simulink subsystem "Map_to_queue"  (R2020a)
settings: Solver=VariableStepAuto  StartTime=0.0  StopTime=10.0  RelTol=1e-3
libraries: simulink x1
settings Model: Creator=zinoex  LastModifiedBy=zinoex

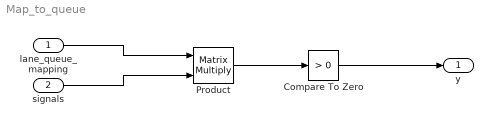
== system Map_to_queue ==
  lane_queue_mapping : Inport
  signals : Inport  Port=2
  Compare To Zero : simulink/Logic and Bit Operations/Compare To Zero  relop=>  OutDataTypeStr=boolean
  Product : Product  Multiplication=Matrix(*)
  y : Outport
  wires:
  signals/1 -> Product/2
  lane_queue_mapping/1 -> Product/1
  Product/1 -> Compare To Zero/1
  Compare To Zero/1 -> y/1
